simulink model "model1"  (R2020a)
settings: Solver=VariableStepAuto  StartTime=0.0  StopTime=10.0  RelTol=1e-3
settings Model: Creator=PRATIKSHA  LastModifiedBy=PRATIKSHA

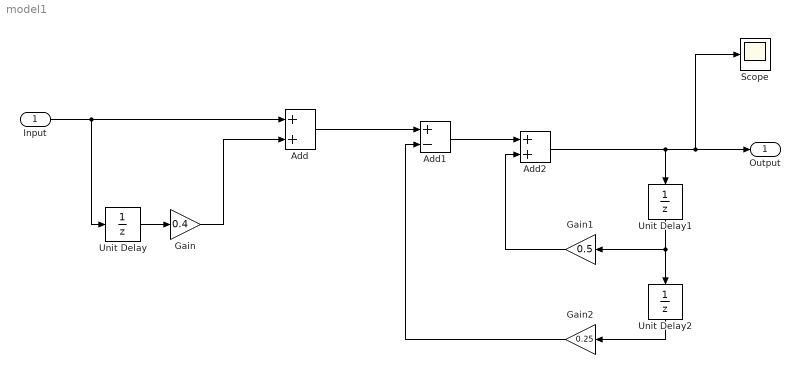
== system model1 ==
  Input : Inport
  Add : Sum
  Add1 : Sum  Inputs=+-
  Add2 : Sum
  Gain : Gain  Gain=0.4
  Gain1 : Gain  Gain=0.5
  Gain2 : Gain  Gain=0.25
  Scope : Scope
  Unit Delay : UnitDelay  SampleTime=-1  HasFrameUpgradeWarning=on
  Unit Delay1 : UnitDelay  SampleTime=-1  HasFrameUpgradeWarning=on
  Unit Delay2 : UnitDelay  SampleTime=-1  HasFrameUpgradeWarning=on
  Output : Outport
  wires:
  Input/1 -> Unit Delay/1, Add/1
  Unit Delay1/1 -> Unit Delay2/1, Gain1/1
  Add2/1 -> Unit Delay1/1, Output/1, Scope/1
  Gain1/1 -> Add2/2
  Gain/1 -> Add/2
  Unit Delay/1 -> Gain/1
  Add1/1 -> Add2/1
  Unit Delay2/1 -> Gain2/1
  Add/1 -> Add1/1
  Gain2/1 -> Add1/2
